simulink model "gm_sampleModel1616_3_sub"  (R2023a)
settings: Solver=VariableStepAuto  StartTime=0.0  StopTime=10.0  RelTol=1e-3
libraries: simulink x1
settings Model: Creator=user1  LastModifiedBy=user1
settings OptimizationCC: BlockReduction=off  ConditionallyExecuteInputs=off
settings DebuggingCC: InheritedTsInSrcMsg=none

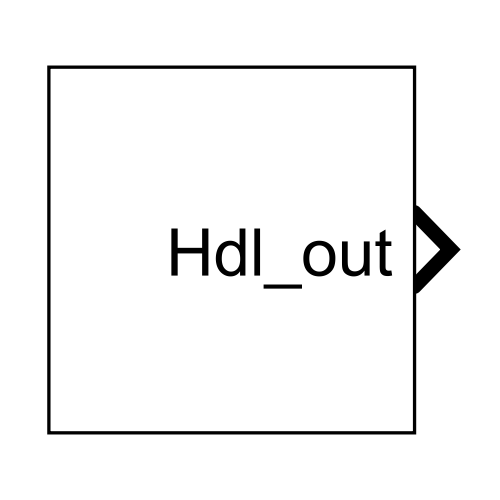
[thumbnail: Simulink's stored preview of the top-level diagram]
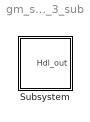
== system gm_sampleModel1616_3_sub ==
  Subsystem : Subsystem

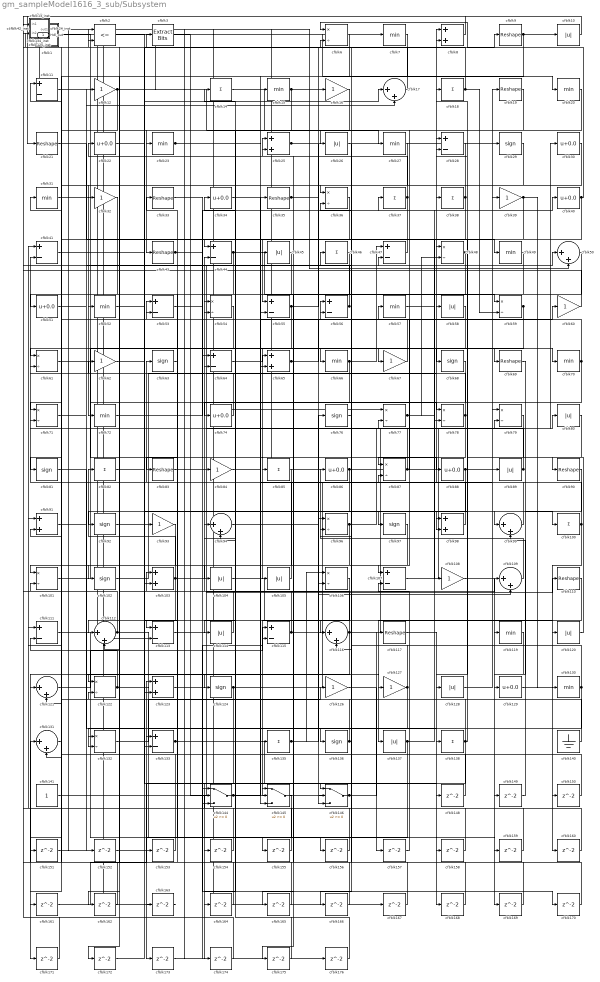
== system gm_sampleModel1616_3_sub/Subsystem ==
  cfblk1 : Subsystem  mask(Compare To Constant){relop=<=, const=double(3), OutDataTypeStr=uint8, ZeroCross=on}
      mask prompts: relop "Simulink:masks:Operator_MP"; const "Simulink:masks:ConstantValue_MP"; OutDataTypeStr "Simulink:masks:OutputDataType_MP"; ZeroCross "Simulink:masks:EnableZerocrossingDetection_MP"
      mask help: Simulink:masks:CompareToConstant_MD
      mask init:
      | OutDataTypeStr = 'uint8';
      | ZeroCross = 'on';
      | blkName = 'sampleModel1616_3_sub/Subsystem/cfblk1';
      | const = double(3);
      | const_str = '3.0';
      | const_val = double(3);
      | relop = '<=';
      | setValue = 'fixdt(0, 8)';
      | str = '<= 3';
      mask TypeOptions relop: == | ~= | < | <= | >= | >
      mask TypeOptions OutDataTypeStr: Simulink:masks:uint8 | Simulink:masks:boolean
      mask Callback ZeroCross: sl('zeroCrossEnable', gcbh);
      mask Display: disp(str)
  cfblk{10,26,45,58,80,89,104..105,114,120,128,137} (12 alike) : Abs  OutDataTypeStr=uint8  SaturateOnIntegerOverflow=off
  cfblk{14,18,37..38,46,82,85,100,135,138} (10 alike) : Sum  Inputs=+  OutDataTypeStr=uint8
  cfblk{6,36,48,54,59,61,71,77..79,87,96,101,106,122,132} (16 alike) : Product  Inputs=*/  OutDataTypeStr=uint8  RndMeth=Zero  SaturateOnIntegerOverflow=on
  cfblk{29,63,68,76,81,92,97,102,124,136} (10 alike) : Signum
  cfblk{8,25,65,91,98,103,123} (7 alike) : Sum  OutDataTypeStr=uint8
  cfblk{11,28,41,44,47,53,55..56,64,107,111,113,115,133} (14 alike) : Sum  Inputs=+-  OutDataTypeStr=uint8
  cfblk{12,16,32,39,60,62,67,84,93,108,126..127} (12 alike) : Gain  OutDataTypeStr=uint8
  cfblk{17,50,94,99,109,112,116,121,131} (9 alike) : Sum  Inputs=|++  OutDataTypeStr=uint8
  cfblk{9,19,21,33,35,43,69,83,90,110,117} (11 alike) : Reshape
  cfblk118_inst : Subsystem
  cfblk{7,15,20,23,27,31,49,52,57,66,70,72,119,130} (14 alike) : MinMax  OutDataTypeStr=uint8
  cfblk125_inst : Subsystem
  cfblk{22,30,34,40,51,74,86,88,129} (9 alike) : Bias  Bias=0.0  SaturateOnIntegerOverflow=off
  cfblk134_inst : Subsystem
  cfblk13_inst : Subsystem
  cfblk140 : Ground
  cfblk141 : Constant  OutDataTypeStr=uint8  SampleTime=-1
  cfblk144 : Switch  OutDataTypeStr=uint8  SaturateOnIntegerOverflow=off  InputSameDT=off
  cfblk145 : Switch  OutDataTypeStr=uint8  SaturateOnIntegerOverflow=off  InputSameDT=off
  cfblk146 : Switch  OutDataTypeStr=uint8  SaturateOnIntegerOverflow=off  InputSameDT=off
  cfblk{148..176} (29 alike) : Delay  SampleTime=1
  cfblk2 : RelationalOperator  Operator=<=  OutDataTypeStr=boolean  InputSameDT=off
  cfblk24_inst : Subsystem
  cfblk3 : simulink/Logic and Bit Operations/Extract Bits  bitsToExtract=Upper half  numBits=8  bitIdxRange=[0 7]  outScalingMode=Preserve fixed-point scaling
      settings: LibrarySourceBlock=|
      | hdlsllib/Logic and Bit
      | Operations/Extract Bits
  cfblk4 : Constant  Value=0  OutDataTypeStr=uint8  SampleTime=1
  cfblk42_inst : Subsystem
  Hdl_out : Outport  OutDataTypeStr=uint8  SampleTime=1
  wires:
  cfblk1/1(y) -> cfblk49/1
  cfblk10/1 -> cfblk21/1
  cfblk100/1 -> cfblk63/1, cfblk160/1
  cfblk101/1 -> cfblk67/1
  cfblk102/1 -> cfblk44/2
  cfblk103/1 -> cfblk112/2, cfblk77/2, cfblk39/1, cfblk82/1
  cfblk104/1 -> cfblk120/1
  cfblk105/1 -> cfblk41/2
  cfblk106/1 -> cfblk145/2
  cfblk107/1 -> cfblk80/1
  cfblk108/1 -> cfblk169/1
  cfblk109/1 -> cfblk86/1
  cfblk11/1 -> cfblk105/1
  cfblk110/1 -> cfblk137/1
  cfblk111/1 -> cfblk155/1
  cfblk112/1 -> cfblk13_inst/1(in1), cfblk159/1
  cfblk113/1 -> cfblk110/1
  cfblk114/1 -> cfblk64/2
  cfblk115/1 -> cfblk8/1, cfblk53/1
  cfblk116/1 -> cfblk28/1, cfblk22/1, cfblk171/1
  cfblk117/1 -> cfblk168/1
  cfblk118_inst/1(out1) -> cfblk89/1, cfblk176/1
  cfblk119/1 -> cfblk149/1
  cfblk12/1 -> cfblk81/1, cfblk26/1
  cfblk120/1 -> cfblk90/1
  cfblk121/1 -> cfblk115/1
  cfblk122/1 -> cfblk111/2, cfblk138/1
  cfblk123/1 -> cfblk58/1
  cfblk124/1 -> cfblk34/1, cfblk79/1, cfblk173/1
  cfblk125_inst/1(out1) -> cfblk16/1
  cfblk126/1 -> cfblk157/1
  cfblk127/1 -> cfblk165/1, cfblk46/1
  cfblk128/1 -> cfblk19/1
  cfblk129/1 -> cfblk150/1
  cfblk13_inst/1(out1) -> cfblk50/2, cfblk113/2, cfblk167/1, cfblk7/1
  cfblk130/1 -> cfblk118_inst/1(in1), cfblk132/2
  cfblk131/1 -> cfblk91/2
  cfblk132/1 -> cfblk126/1
  cfblk133/1 -> cfblk35/1, cfblk148/1
  cfblk134_inst/1(out1) -> cfblk77/1, cfblk152/1
  cfblk135/1 -> cfblk76/1, cfblk106/1
  cfblk136/1 -> cfblk111/1, cfblk96/2
  cfblk137/1 -> cfblk40/1, cfblk163/1
  cfblk138/1 -> cfblk25/1, cfblk174/1, cfblk18/1
  cfblk14/1 -> cfblk27/1
  cfblk140/1 -> cfblk96/1
  cfblk141/1 -> cfblk109/1
  cfblk144/1 -> cfblk87/2, cfblk37/1
  cfblk145/1 -> cfblk154/1
  cfblk146/1 -> cfblk117/1, Hdl_out/1
  cfblk148/1 -> cfblk103/1
  cfblk149/1 -> cfblk99/2
  cfblk15/1 -> cfblk92/1, cfblk43/1
  cfblk150/1 -> cfblk101/2
  cfblk151/1 -> cfblk17/2
  cfblk152/1 -> cfblk123/1
  cfblk153/1 -> cfblk118_inst/2(in2)
  cfblk154/1 -> cfblk125_inst/2(in2)
  cfblk155/1 -> cfblk41/1
  cfblk156/1 -> cfblk54/1
  cfblk157/1 -> cfblk107/2
  cfblk158/1 -> cfblk11/1
  cfblk159/1 -> cfblk36/2
  cfblk16/1 -> cfblk23/1
  cfblk160/1 -> cfblk91/1
  cfblk161/1 -> cfblk133/1
  cfblk162/1 -> cfblk131/1
  cfblk163/1 -> cfblk1/1(u)
  cfblk164/1 -> cfblk13_inst/2(in2)
  cfblk165/1 -> cfblk2/1
  cfblk166/1 -> cfblk121/2
  cfblk167/1 -> cfblk25/2
  cfblk168/1 -> cfblk56/1
  cfblk169/1 -> cfblk53/2
  cfblk17/1 -> cfblk125_inst/1(in1)
  cfblk170/1 -> cfblk122/2
  cfblk171/1 -> cfblk24_inst/2(in2)
  cfblk172/1 -> cfblk48/1
  cfblk173/1 -> cfblk115/2
  cfblk174/1 -> cfblk134_inst/2(in2)
  cfblk175/1 -> cfblk94/1
  cfblk176/1 -> cfblk144/2
  cfblk18/1 -> cfblk3/1, cfblk59/2
  cfblk19/1 -> cfblk87/1
  cfblk2/1 -> cfblk103/2
  cfblk20/1 -> cfblk74/1
  cfblk21/1 -> cfblk44/1
  cfblk22/1 -> cfblk146/1
  cfblk23/1 -> cfblk68/1, cfblk55/2
  cfblk24_inst/1(out1) -> cfblk15/1
  cfblk25/1 -> cfblk146/2, cfblk59/1
  cfblk26/1 -> cfblk66/1
  cfblk27/1 -> cfblk72/1
  cfblk28/1 -> cfblk61/1
  cfblk29/1 -> cfblk132/1
  cfblk3/1 -> cfblk20/1
  cfblk30/1 -> cfblk166/1
  cfblk31/1 -> cfblk123/2
  cfblk32/1 -> cfblk51/1
  cfblk33/1 -> cfblk64/1
  cfblk34/1 -> cfblk136/1
  cfblk35/1 -> cfblk69/1, cfblk78/1
  cfblk36/1 -> cfblk121/1
  cfblk37/1 -> cfblk55/1, cfblk2/2
  cfblk38/1 -> cfblk145/3, cfblk78/2, cfblk36/1
  cfblk39/1 -> cfblk98/2, cfblk130/1
  cfblk4/1 -> cfblk11/2
  cfblk40/1 -> cfblk6/1, cfblk52/1
  cfblk41/1 -> cfblk99/1
  cfblk42_inst/1(out1) -> cfblk29/1
  cfblk43/1 -> cfblk88/1, cfblk170/1, cfblk158/1
  cfblk44/1 -> cfblk146/3, cfblk112/1
  cfblk45/1 -> cfblk114/1
  cfblk46/1 -> cfblk83/1
  cfblk47/1 -> cfblk45/1
  cfblk48/1 -> cfblk145/1, cfblk71/1, cfblk122/1
  cfblk49/1 -> cfblk144/3
  cfblk50/1 -> cfblk153/1
  cfblk51/1 -> cfblk12/1
  cfblk52/1 -> cfblk93/1
  cfblk53/1 -> cfblk144/1
  cfblk54/1 -> cfblk101/1
  cfblk55/1 -> cfblk8/2, cfblk85/1
  cfblk56/1 -> cfblk42_inst/1(in1), cfblk24_inst/1(in1)
  cfblk57/1 -> cfblk70/1
  cfblk58/1 -> cfblk131/2
  cfblk59/1 -> cfblk124/1, cfblk106/2
  cfblk6/1 -> cfblk161/1
  cfblk60/1 -> cfblk42_inst/2(in2)
  cfblk61/1 -> cfblk108/1
  cfblk62/1 -> cfblk17/1
  cfblk63/1 -> cfblk113/1
  cfblk64/1 -> cfblk65/1
  cfblk65/1 -> cfblk60/1, cfblk100/1
  cfblk66/1 -> cfblk47/1, cfblk164/1
  cfblk67/1 -> cfblk31/1
  cfblk68/1 -> cfblk97/1
  cfblk69/1 -> cfblk119/1
  cfblk7/1 -> cfblk32/1
  cfblk70/1 -> cfblk94/2, cfblk6/2
  cfblk71/1 -> cfblk47/2
  cfblk72/1 -> cfblk38/1
  cfblk74/1 -> cfblk33/1
  cfblk76/1 -> cfblk156/1
  cfblk77/1 -> cfblk50/1, cfblk48/2
  cfblk78/1 -> cfblk107/1, cfblk61/2
  cfblk79/1 -> cfblk98/1
  cfblk8/1 -> cfblk134_inst/1(in1)
  cfblk80/1 -> cfblk128/1
  cfblk81/1 -> cfblk127/1
  cfblk82/1 -> cfblk9/1
  cfblk83/1 -> cfblk30/1
  cfblk84/1 -> cfblk56/2
  cfblk85/1 -> cfblk151/1
  cfblk86/1 -> cfblk116/2, cfblk175/1
  cfblk87/1 -> cfblk62/1, cfblk57/1
  cfblk88/1 -> cfblk28/2, cfblk102/1
  cfblk89/1 -> cfblk71/2, cfblk54/2
  cfblk9/1 -> cfblk65/2, cfblk10/1
  cfblk90/1 -> cfblk129/1
  cfblk91/1 -> cfblk133/2
  cfblk92/1 -> cfblk116/1
  cfblk93/1 -> cfblk162/1
  cfblk94/1 -> cfblk109/2
  cfblk96/1 -> cfblk79/2, cfblk172/1, cfblk135/1
  cfblk97/1 -> cfblk104/1
  cfblk98/1 -> cfblk84/1
  cfblk99/1 -> cfblk14/1

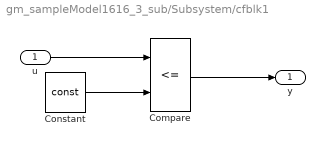
== system gm_sampleModel1616_3_sub/Subsystem/cfblk1 ==
  u : Inport  OutDataTypeStr=uint8  SampleTime=1
  Compare : RelationalOperator  Operator=<=  OutDataTypeStr=fixdt(0, 8)
  Constant : Constant  DisableCoverage=on  Value=const  OutDataTypeStr=Inherit: Inherit via back propagation  SampleTime=-1
  y : Outport  SampleTime=1
  wires:
  u/1 -> Compare/1
  Compare/1 -> y/1
  Constant/1 -> Compare/2

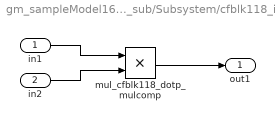
== system gm_sampleModel1616_3_sub/Subsystem/cfblk118_inst ==
  in1 : Inport  OutDataTypeStr=uint8  SampleTime=1
  in2 : Inport  Port=2  OutDataTypeStr=uint8  SampleTime=1
  mul_cfblk118_dotp_mulcomp : Product  Inputs=**  OutDataTypeStr=uint8  SampleTime=1
  out1 : Outport  OutDataTypeStr=uint8  SampleTime=1
  wires:
  in1/1 -> mul_cfblk118_dotp_mulcomp/1
  in2/1 -> mul_cfblk118_dotp_mulcomp/2
  mul_cfblk118_dotp_mulcomp/1 -> out1/1

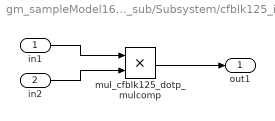
== system gm_sampleModel1616_3_sub/Subsystem/cfblk125_inst ==
  in1 : Inport  OutDataTypeStr=uint8  SampleTime=1
  in2 : Inport  Port=2  OutDataTypeStr=uint8  SampleTime=1
  mul_cfblk125_dotp_mulcomp : Product  Inputs=**  OutDataTypeStr=uint8  SampleTime=1
  out1 : Outport  OutDataTypeStr=uint8  SampleTime=1
  wires:
  in1/1 -> mul_cfblk125_dotp_mulcomp/1
  in2/1 -> mul_cfblk125_dotp_mulcomp/2
  mul_cfblk125_dotp_mulcomp/1 -> out1/1

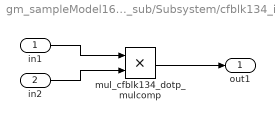
== system gm_sampleModel1616_3_sub/Subsystem/cfblk134_inst ==
  in1 : Inport  OutDataTypeStr=uint8  SampleTime=1
  in2 : Inport  Port=2  OutDataTypeStr=uint8  SampleTime=1
  mul_cfblk134_dotp_mulcomp : Product  Inputs=**  OutDataTypeStr=uint8  SampleTime=1
  out1 : Outport  OutDataTypeStr=uint8  SampleTime=1
  wires:
  in1/1 -> mul_cfblk134_dotp_mulcomp/1
  in2/1 -> mul_cfblk134_dotp_mulcomp/2
  mul_cfblk134_dotp_mulcomp/1 -> out1/1

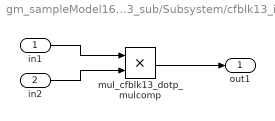
== system gm_sampleModel1616_3_sub/Subsystem/cfblk13_inst ==
  in1 : Inport  OutDataTypeStr=uint8  SampleTime=1
  in2 : Inport  Port=2  OutDataTypeStr=uint8  SampleTime=1
  mul_cfblk13_dotp_mulcomp : Product  Inputs=**  OutDataTypeStr=uint8  SampleTime=1
  out1 : Outport  OutDataTypeStr=uint8  SampleTime=1
  wires:
  in1/1 -> mul_cfblk13_dotp_mulcomp/1
  in2/1 -> mul_cfblk13_dotp_mulcomp/2
  mul_cfblk13_dotp_mulcomp/1 -> out1/1

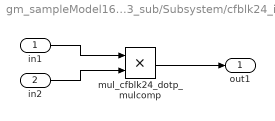
== system gm_sampleModel1616_3_sub/Subsystem/cfblk24_inst ==
  in1 : Inport  OutDataTypeStr=uint8  SampleTime=1
  in2 : Inport  Port=2  OutDataTypeStr=uint8  SampleTime=1
  mul_cfblk24_dotp_mulcomp : Product  Inputs=**  OutDataTypeStr=uint8  SampleTime=1
  out1 : Outport  OutDataTypeStr=uint8  SampleTime=1
  wires:
  in1/1 -> mul_cfblk24_dotp_mulcomp/1
  in2/1 -> mul_cfblk24_dotp_mulcomp/2
  mul_cfblk24_dotp_mulcomp/1 -> out1/1

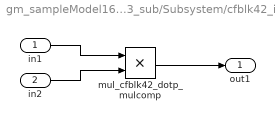
== system gm_sampleModel1616_3_sub/Subsystem/cfblk42_inst ==
  in1 : Inport  OutDataTypeStr=uint8  SampleTime=1
  in2 : Inport  Port=2  OutDataTypeStr=uint8  SampleTime=1
  mul_cfblk42_dotp_mulcomp : Product  Inputs=**  OutDataTypeStr=uint8  SampleTime=1
  out1 : Outport  OutDataTypeStr=uint8  SampleTime=1
  wires:
  in1/1 -> mul_cfblk42_dotp_mulcomp/1
  in2/1 -> mul_cfblk42_dotp_mulcomp/2
  mul_cfblk42_dotp_mulcomp/1 -> out1/1
